simulink model "DACS"  (R2022b)
settings: Solver=VariableStepAuto  StartTime=0.0  StopTime=10  RelTol=1e-3
InitFcn:
  | DACSpara
values from neighbouring files (symbols this model uses):
  Amax = 362.97    [DACSpara.m]
  Dmax = 5415.1    [DACSpara.m]
  g = 9.52    [DACSpara.m]
  Ixx = M*(ly^2)/2    (= 0.2997)    [DACSpara.m]
  Iyy = M*(3*ly^2+4*lx^2)/12    (= 82.3052666667)    [DACSpara.m]
  Izz = M*(3*ly^2+4*lx^2)/12    (= 82.3052666667)    [DACSpara.m]
  Kd = 400    [Controlgain.m]    (also in DACSpara.m)
  Kp = 600    [Controlgain.m]    (also in DACSpara.m)
  Kp1 = 600    [Controlgain.m]    (also in DACSpara.m)
  Kp2 = 150    [Controlgain.m]    (also in DACSpara.m)
  lx = 1.825    [DACSpara.m]
  ly = 0.09    [DACSpara.m]
  M = 74    [DACSpara.m]
  N = 3    [Controlgain.m]    (also in DACSpara.m = 5)
  POSinit = [0; 0; 0]    [DACSpara.m]
  PQRinit = [0; 0; 0]    [DACSpara.m]
  Quatinit = Euler2Quat([phi;theta;psi].*d2r)    [DACSpara.m]
  Theading = Euler2Quat([0;-30;180].*d2r)    [DACSpara.m]
  TPosition = 20000*[Tpos(2);Tpos(3);-Tpos(4)]    [DACSpara.m]    (also in Targetpara.m = Tdist*[Tpos(2);Tpos(3);-Tpos(4)])
  Tspeed = 2500    [DACSpara.m]
  UVWinit = [1000; 0; 0]    [DACSpara.m]
libraries: matrix_library x2, dspmtrx3 x1, uavutilslib x1
settings Model: PacingRate=0.010000  Creator=tn  LastModifiedBy=tn
settings DataIOCC: ReturnWorkspaceOutputs=off

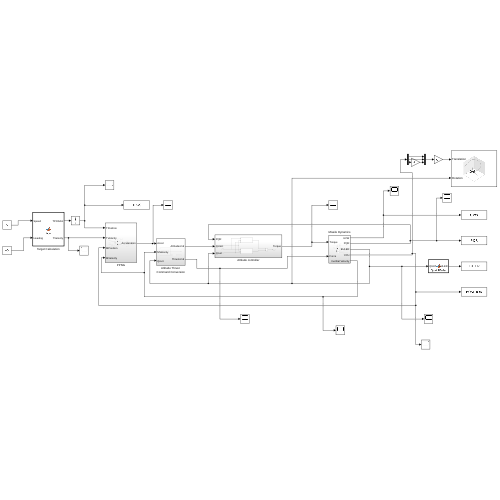
[thumbnail: Simulink's stored preview of the top-level diagram]
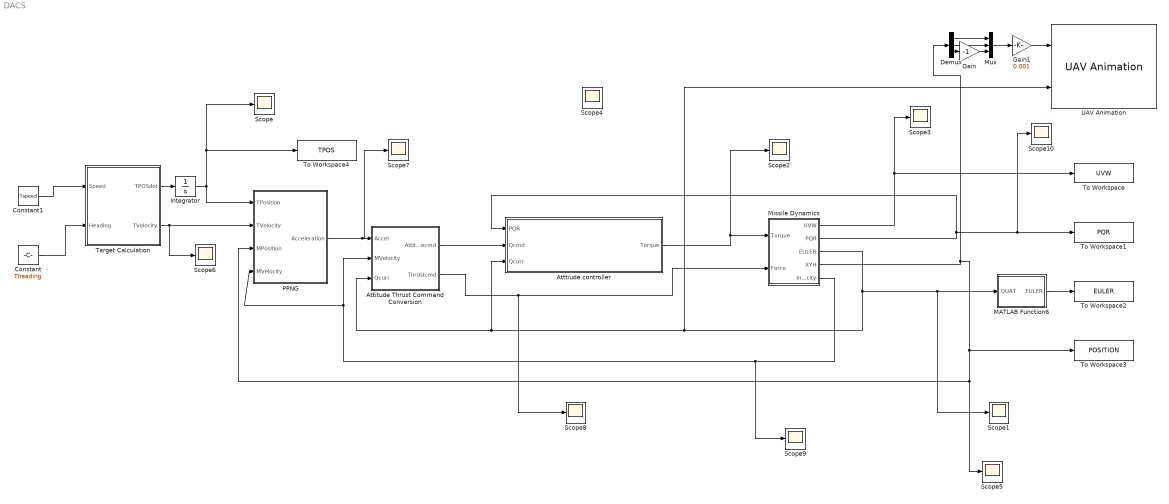
== system DACS ==
  Attitude Thrust Command Conversion : Subsystem
  Atttiude controller : Subsystem
  Constant : Constant  Value=Theading
  Constant1 : Constant  Value=Tspeed
  Demux : Demux  Outputs=3
  Gain : Gain  Gain=-1
  Gain1 : Gain  Gain=0.001
  Integrator : Integrator  InitialCondition=TPosition
  MATLAB Function6 : MATLAB Function  TreatAsAtomicUnit=on
  Missile Dynamics : Subsystem
  Mux : Mux  Inputs=3
  PPNG : Subsystem
  Scope{,1..10} (11 alike) : Scope
  Target Calculation : MATLAB Function  TreatAsAtomicUnit=on
  To Workspace : ToWorkspace  VariableName=UVW  SaveFormat=Timeseries  SampleTime=-1
  To Workspace1 : ToWorkspace  VariableName=PQR  SaveFormat=Timeseries  SampleTime=-1
  To Workspace2 : ToWorkspace  VariableName=EULER  SaveFormat=Timeseries  SampleTime=-1
  To Workspace3 : ToWorkspace  VariableName=POSITION  SaveFormat=Timeseries  SampleTime=-1
  To Workspace4 : ToWorkspace  VariableName=TPOS  SaveFormat=Timeseries  SampleTime=-1
  UAV Animation : uavutilslib/UAV Animation  UAVType=FixedWing  UAVSize=1  InertialZDirection=Down  SampleTime=-1
  wires:
  Missile Dynamics/1(UVW) -> To Workspace/1, Scope3/1
  Missile Dynamics/4(XYH) -> Demux/1, Scope5/1, PPNG/3(MPosition), To Workspace3/1
  Missile Dynamics/2(PQR) -> Atttiude controller/1(PQR), Scope10/1, To Workspace1/1
  Atttiude controller/1(Torque) -> Scope2/1, Missile Dynamics/1(Torque)
  Missile Dynamics/3(EULER) -> Atttiude controller/3(Qcurr), Attitude Thrust Command Conversion/3(Qcurr), UAV Animation/2, MATLAB Function6/1(QUAT), Scope1/1
  Missile Dynamics/5(Inerttial Velocity) -> Scope9/1, Attitude Thrust Command Conversion/2(MVelocity), PPNG/4(MVelocity)
  PPNG/1(Acceleration) -> Scope7/1, Attitude Thrust Command Conversion/1(Accel)
  Attitude Thrust Command Conversion/1(Attitudecmd) -> Atttiude controller/2(Qcmd)
  MATLAB Function6/1(EULER) -> To Workspace2/1
  Attitude Thrust Command Conversion/2(Thrustcmd) -> Scope8/1, Missile Dynamics/2(Force)
  Target Calculation/2(TVelocity) -> Scope6/1, PPNG/2(TVelocity)
  Integrator/1 -> Scope/1, To Workspace4/1, PPNG/1(TPosition)
  Constant1/1 -> Target Calculation/1(Speed)
  Constant/1 -> Target Calculation/2(Heading)
  Demux/1 -> Mux/1
  Demux/2 -> Mux/2
  Demux/3 -> Gain/1
  Gain/1 -> Mux/3
  Target Calculation/1(TPOSdot) -> Integrator/1
  Mux/1 -> Gain1/1
  Gain1/1 -> UAV Animation/1

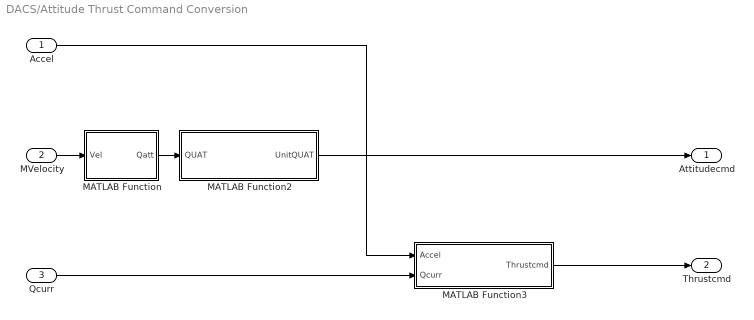
== system DACS/Attitude Thrust Command Conversion ==
  Accel : Inport
  MVelocity : Inport  Port=2
  Qcurr : Inport  Port=3
  MATLAB Function : MATLAB Function  TreatAsAtomicUnit=on
  MATLAB Function2 : MATLAB Function  TreatAsAtomicUnit=on
  MATLAB Function3 : MATLAB Function  TreatAsAtomicUnit=on
  Attitudecmd : Outport
  Thrustcmd : Outport  Port=2
  wires:
  MATLAB Function/1(Qatt) -> MATLAB Function2/1(QUAT)
  MVelocity/1 -> MATLAB Function/1(Vel)
  MATLAB Function2/1(UnitQUAT) -> Attitudecmd/1
  Qcurr/1 -> MATLAB Function3/2(Qcurr)
  Accel/1 -> MATLAB Function3/1(Accel)
  MATLAB Function3/1(Thrustcmd) -> Thrustcmd/1

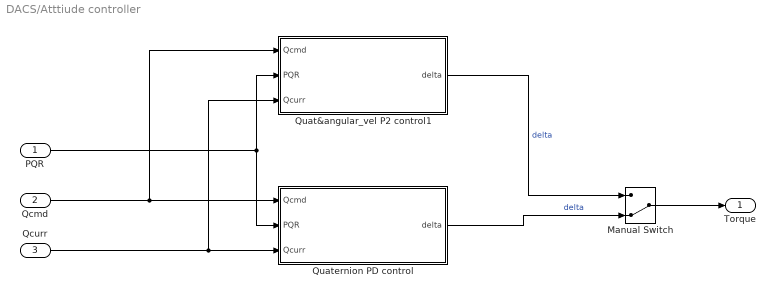
== system DACS/Atttiude controller ==
  PQR : Inport
  Qcmd : Inport  Port=2
  Qcurr : Inport  Port=3
  Manual Switch : ManualSwitch  CurrentSetting=0
  Quat&angular_vel P2 control1 : Subsystem
  Quaternion PD control : Subsystem
  Torque : Outport
  wires:
  Quaternion PD control/1(delta) -> Manual Switch/2  "delta"
  Quat&angular_vel P2 control1/1(delta) -> Manual Switch/1  "delta"
  Qcurr/1 -> Quaternion PD control/3(Qcurr), Quat&angular_vel P2 control1/3(Qcurr)
  Manual Switch/1 -> Torque/1
  Qcmd/1 -> Quaternion PD control/1(Qcmd), Quat&angular_vel P2 control1/1(Qcmd)
  PQR/1 -> Quat&angular_vel P2 control1/2(PQR), Quaternion PD control/2(PQR)

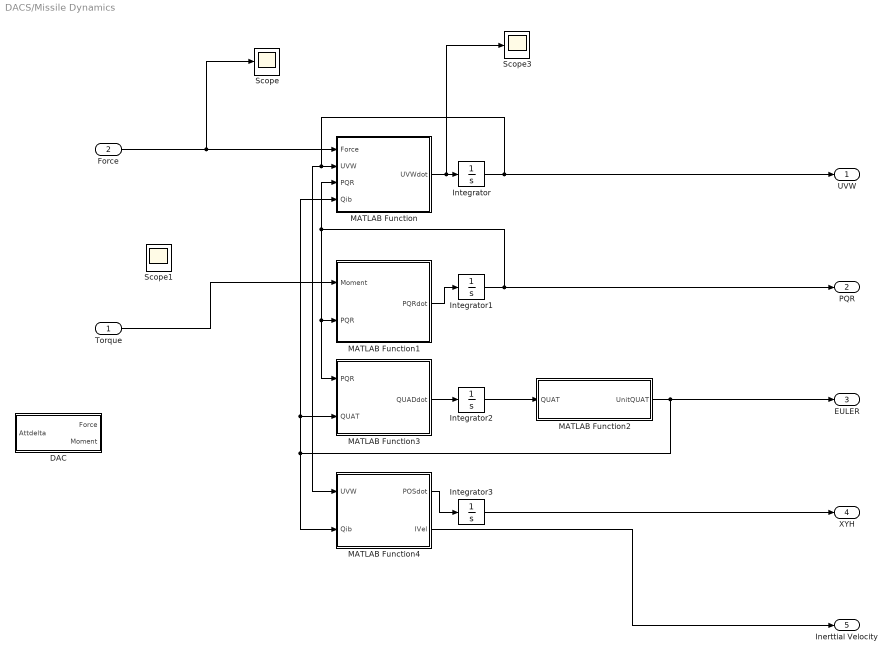
== system DACS/Missile Dynamics ==
  Torque : Inport
  Force : Inport  Port=2
  DAC : Subsystem
  Integrator : Integrator  InitialCondition=UVWinit
  Integrator1 : Integrator  InitialCondition=PQRinit
  Integrator2 : Integrator  InitialCondition=Quatinit
  Integrator3 : Integrator  InitialCondition=POSinit
  MATLAB Function : MATLAB Function  TreatAsAtomicUnit=on
  MATLAB Function1 : MATLAB Function  TreatAsAtomicUnit=on
  MATLAB Function2 : MATLAB Function  TreatAsAtomicUnit=on
  MATLAB Function3 : MATLAB Function  TreatAsAtomicUnit=on
  MATLAB Function4 : MATLAB Function  TreatAsAtomicUnit=on
  Scope : Scope
  Scope1 : Scope
  Scope3 : Scope
  UVW : Outport
  PQR : Outport  Port=2
  EULER : Outport  Port=3
  XYH : Outport  Port=4
  Inerttial Velocity : Outport  Port=5
  wires:
  MATLAB Function/1(UVWdot) -> Scope3/1, Integrator/1
  MATLAB Function1/1(PQRdot) -> Integrator1/1
  MATLAB Function3/1(QUADdot) -> Integrator2/1
  MATLAB Function4/1(POSdot) -> Integrator3/1
  Integrator/1 -> UVW/1, MATLAB Function4/1(UVW), MATLAB Function/2(UVW)
  Integrator1/1 -> PQR/1, MATLAB Function3/1(PQR), MATLAB Function1/2(PQR), MATLAB Function/3(PQR)
  Integrator2/1 -> MATLAB Function2/1(QUAT)
  MATLAB Function2/1(UnitQUAT) -> EULER/1, MATLAB Function4/2(Qib), MATLAB Function/4(Qib), MATLAB Function3/2(QUAT)
  Integrator3/1 -> XYH/1
  Torque/1 -> MATLAB Function1/1(Moment)
  Force/1 -> Scope/1, MATLAB Function/1(Force)
  MATLAB Function4/2(IVel) -> Inerttial Velocity/1

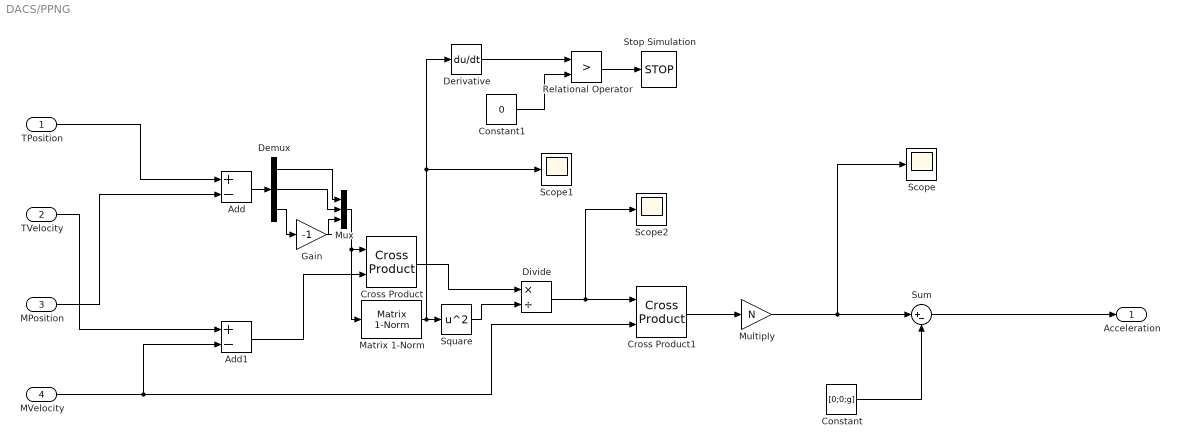
== system DACS/PPNG ==
  TPosition : Inport
  TVelocity : Inport  Port=2
  MPosition : Inport  Port=3
  MVelocity : Inport  Port=4
  Add : Sum  Inputs=+-
  Add1 : Sum  Inputs=+-
  Constant : Constant  Value=[0;0;g]
  Constant1 : Constant  Value=0
  Cross Product : matrix_library/Cross Product
  Cross Product1 : matrix_library/Cross Product
  Demux : Demux  Outputs=3
  Derivative : Derivative
  Divide : Product  Inputs=*/
  Gain : Gain  Gain=-1
  Matrix 1-Norm : dspmtrx3/Matrix  1-Norm  roundingMode=Floor  overflowMode=off  outputDataTypeStr=Inherit: Same as accumulator  outputMin=[]  outputMax=[]  outputLastDataTypeStr=Inherit: Same as accumulator
  Multiply : Gain  Gain=N
  Mux : Mux  Inputs=3
  Relational Operator : RelationalOperator  Operator=>  OutDataTypeStr=boolean  RndMeth=Simplest  InputSameDT=off
  Scope : Scope
  Scope1 : Scope
  Scope2 : Scope
  Square : Math  Operator=square
  Stop Simulation : Stop
  Sum : Sum  Inputs=|+-
  Acceleration : Outport
  wires:
  MPosition/1 -> Add/2
  TVelocity/1 -> Add1/1
  MVelocity/1 -> Cross Product1/2, Add1/2
  Add/1 -> Demux/1
  Add1/1 -> Cross Product/2
  Cross Product/1 -> Divide/1
  Divide/1 -> Scope2/1, Cross Product1/1
  Cross Product1/1 -> Multiply/1
  Multiply/1 -> Scope/1, Sum/1
  Constant/1 -> Sum/2
  Sum/1 -> Acceleration/1
  Square/1 -> Divide/2
  Matrix 1-Norm/1 -> Derivative/1, Scope1/1, Square/1
  Demux/3 -> Gain/1
  Constant1/1 -> Relational Operator/2
  TPosition/1 -> Add/1
  Demux/1 -> Mux/1
  Demux/2 -> Mux/2
  Gain/1 -> Mux/3
  Mux/1 -> Matrix 1-Norm/1, Cross Product/1
  Derivative/1 -> Relational Operator/1
  Relational Operator/1 -> Stop Simulation/1

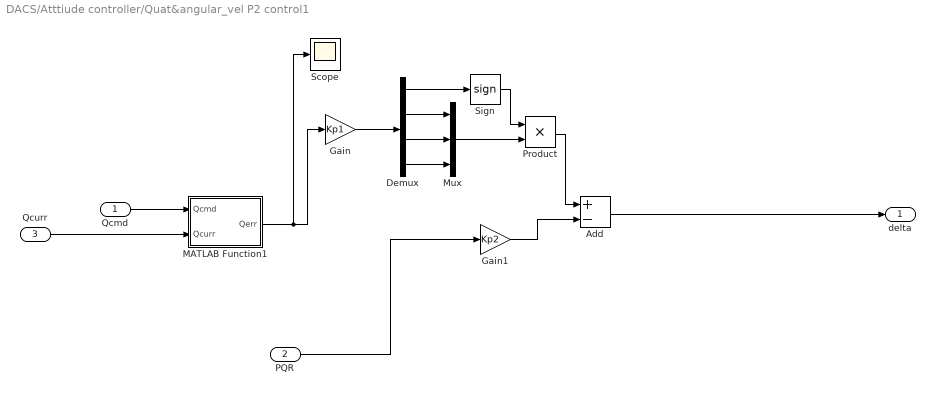
== system DACS/Atttiude controller/Quat&angular_vel P2 control1 ==
  Qcmd : Inport
  PQR : Inport  Port=2
  Qcurr : Inport  Port=3
  Add : Sum  Inputs=+-
  Demux : Demux
  Gain : Gain  Gain=Kp1
  Gain1 : Gain  Gain=Kp2
  MATLAB Function1 : MATLAB Function  TreatAsAtomicUnit=on
  Mux : Mux  Inputs=3
  Product : Product
  Scope : Scope
  Sign : Signum
  delta : Outport
  wires:
  Demux/3 -> Mux/2
  Demux/2 -> Mux/1
  MATLAB Function1/1(Qerr) -> Scope/1, Gain/1
  Gain1/1 -> Add/2
  PQR/1 -> Gain1/1
  Demux/4 -> Mux/3
  Qcurr/1 -> MATLAB Function1/2(Qcurr)
  Qcmd/1 -> MATLAB Function1/1(Qcmd)
  Gain/1 -> Demux/1
  Add/1 -> delta/1
  Demux/1 -> Sign/1
  Mux/1 -> Product/2
  Sign/1 -> Product/1
  Product/1 -> Add/1

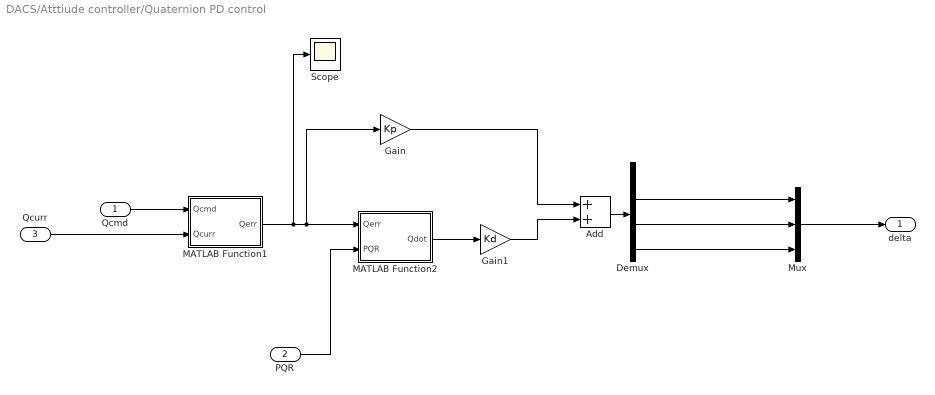
== system DACS/Atttiude controller/Quaternion PD control ==
  Qcmd : Inport
  PQR : Inport  Port=2
  Qcurr : Inport  Port=3
  Add : Sum
  Demux : Demux
  Gain : Gain  Gain=Kp
  Gain1 : Gain  Gain=Kd
  MATLAB Function1 : MATLAB Function  TreatAsAtomicUnit=on
  MATLAB Function2 : MATLAB Function  TreatAsAtomicUnit=on
  Mux : Mux  Inputs=3
  Scope : Scope
  delta : Outport
  wires:
  Demux/3 -> Mux/2
  PQR/1 -> MATLAB Function2/2(PQR)
  Demux/2 -> Mux/1
  Gain/1 -> Add/1
  MATLAB Function1/1(Qerr) -> Scope/1, Gain/1, MATLAB Function2/1(Qerr)
  Gain1/1 -> Add/2
  Add/1 -> Demux/1
  MATLAB Function2/1(Qdot) -> Gain1/1
  Demux/4 -> Mux/3
  Qcurr/1 -> MATLAB Function1/2(Qcurr)
  Qcmd/1 -> MATLAB Function1/1(Qcmd)
  Mux/1 -> delta/1

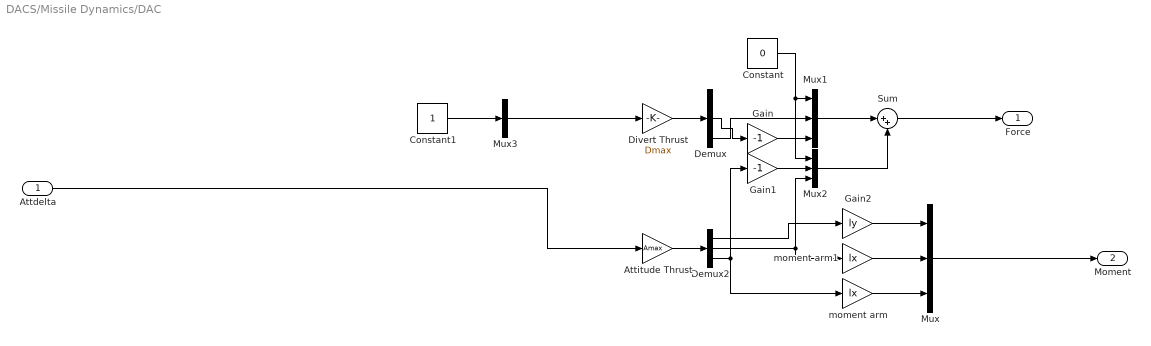
== system DACS/Missile Dynamics/DAC ==
  Attdelta : Inport
  Attitude Thrust : Gain  Gain=Amax
  Constant : Constant  Value=0
  Constant1 : Constant
  Demux : Demux  Outputs=3
  Demux2 : Demux  Outputs=3
  Divert Thrust : Gain  Gain=Dmax
  Gain : Gain  Gain=-1
  Gain1 : Gain  Gain=-1
  Gain2 : Gain  Gain=ly
  Mux{,1..3} (4 alike) : Mux  Inputs=3
  Sum : Sum  Inputs=|++
  moment arm : Gain  Gain=lx
  moment arm1 : Gain  Gain=lx
  Force : Outport
  Moment : Outport  Port=2
  wires:
  Attitude Thrust/1 -> Demux2/1
  Sum/1 -> Force/1
  Mux1/1 -> Sum/1
  Demux2/1 -> Gain2/1
  Gain/1 -> Mux1/3
  Demux2/3 -> moment arm/1, Gain1/1
  Gain1/1 -> Mux2/2
  Demux2/2 -> moment arm1/1, Mux2/3
  Mux2/1 -> Sum/2
  Mux/1 -> Moment/1
  Constant/1 -> Mux1/1, Mux2/1
  Divert Thrust/1 -> Demux/1
  Demux/3 -> Mux1/2
  Demux/2 -> Gain/1
  Gain2/1 -> Mux/1
  moment arm1/1 -> Mux/2
  moment arm/1 -> Mux/3
  Attdelta/1 -> Attitude Thrust/1
  Constant1/1 -> Mux3/2
  Mux3/1 -> Divert Thrust/1

== matlab function DACS/Attitude Thrust Command Conversion/MATLAB Function ==
  data: Vel input; Qatt output
function Qatt = fcn(Vel)

if (nnz(Vel./norm(Vel) == -[1;0;0]) == 3)
    Qatt = [0;0;1;0];
    return
end

temp = cross([1;0;0],Vel);
q0 = norm(Vel)+dot(Vel,[1;0;0]);

Qatt = [q0;temp(1);temp(2);temp(3)];
end

== matlab function DACS/Attitude Thrust Command Conversion/MATLAB Function3 ==
  data: Accel input; Thrustcmd output; Qcurr input; Dmax parameter; M parameter
function Thrustcmd   = Projection(Accel, Qcurr, Dmax,M)

temp = Quatmul(Quatmul(Quatinv(Qcurr),Accel),Qcurr);
Thrustcmd = M.*[0;temp(3);temp(4)];
if (norm(Thrustcmd) > Dmax)
    Thrustcmd = Dmax*Thrustcmd./norm(Thrustcmd);
end

== matlab function DACS/Attitude Thrust Command Conversion/MATLAB Function2 ==
  data: QUAT input; UnitQUAT output
function UnitQUAT = NormalizeQuat(QUAT)

q0 = QUAT(1);
q1 = QUAT(2);
q2 = QUAT(3);
q3 = QUAT(4);

Qabs = sqrt(q0^2+q1^2+q2^2+q3^2);

q0 = q0/Qabs;
q1 = q1/Qabs;
q2 = q2/Qabs;
q3 = q3/Qabs;

UnitQUAT = [q0;q1;q2;q3];
end

== matlab function DACS/Missile Dynamics/MATLAB Function1 ==
  data: Moment input; PQRdot output; PQR input; Ixx parameter; Iyy parameter; Izz parameter
function PQRdot = PQR_dot(Moment, PQR, Ixx, Iyy, Izz)

p = PQR(1);
q = PQR(2);
r = PQR(3);

% L=0, So p_dot is zero, p is constant value
L = Moment(1);
M = Moment(2);
N = Moment(3);

p_dot = L/Ixx - (Izz-Iyy)*q*r/Ixx;
q_dot = M/Iyy - (Ixx-Izz)*p*r/Iyy;
r_dot = N/Izz - (Iyy-Ixx)*p*q/Izz;

PQRdot = [p_dot;q_dot;r_dot];

== matlab function DACS/Missile Dynamics/MATLAB Function ==
  data: Force input; UVWdot output; UVW input; PQR input; Qib input; M parameter
function UVWdot= UVW_dot(Force,UVW,PQR,Qib,M)

g=9.52;   % gravity @ 100km height [m/s^2]

fx = Force(1);
fy = Force(2);
fz = Force(3);

u = UVW(1);
v = UVW(2);
w = UVW(3);

p = PQR(1);
q = PQR(2);
r = PQR(3);

%gb = Cib'*[0; 0; g];
gcal = Quatmul(Quatmul(Quatinv(Qib),[0;0;g]), Qib);
gb = [gcal(2);gcal(3);gcal(4)];

u_dot = v*r - w*q + fx/M + gb(1);
v_dot = -u*r + w*p + fy/M + gb(2);
w_dot = u*q - v*p + fz/M + gb(3);

UVWdot =[u_dot; v_dot; w_dot];

== matlab function DACS/Missile Dynamics/MATLAB Function3 ==
  data: PQR input; QUAT input; QUADdot output
function QUADdot = QUAT_dot(PQR,QUAT)

q0 = QUAT(1);
q1 = QUAT(2);
q2 = QUAT(3);
q3 = QUAT(4);

p = PQR(1);
q = PQR(2);
r = PQR(3);
    
q0_dot = -1/2*(q1*p +q2*q + q3*r);
q1_dot = 1/2*(q0*p +q2*r - q3*q);
q2_dot = 1/2*(q0*q +q3*p - q1*r);
q3_dot = 1/2*(q0*r +q1*q - q2*p);

QUADdot =[q0_dot; q1_dot; q2_dot; q3_dot];

== matlab function DACS/Missile Dynamics/MATLAB Function4 ==
  data: POSdot output; IVel output; UVW input; Qib input
function [POSdot, IVel] = POS_dot(UVW,Qib)

u = UVW(1);
v = UVW(2);
w = UVW(3);

POSdotcal = Quatmul(Quatmul(Qib,[u; v; w]), Quatinv(Qib));
IVel = [POSdotcal(2);POSdotcal(3);POSdotcal(4)];
POSdot = [1 0 0;0 1 0;0 0 -1]*IVel; % pos=[x,y,h]'

== matlab function DACS/Missile Dynamics/MATLAB Function2 ==
  data: QUAT input; UnitQUAT output
function UnitQUAT = NormalizeQuat(QUAT)

q0 = QUAT(1);
q1 = QUAT(2);
q2 = QUAT(3);
q3 = QUAT(4);

Qabs = sqrt(q0^2+q1^2+q2^2+q3^2);

q0 = q0/Qabs;
q1 = q1/Qabs;
q2 = q2/Qabs;
q3 = q3/Qabs;

UnitQUAT = [q0;q1;q2;q3];
end

== matlab function DACS/Atttiude controller/Quat&angular_vel P2 control1/MATLAB Function1 ==
  data: Qcmd input; Qerr output; Qcurr input
function Qerr = ErrorQ(Qcmd, Qcurr)

qx = Quatinv(Qcurr);

Qerr = Quatmul(qx, Qcmd);
end

== matlab function DACS/MATLAB Function6 ==
  data: QUAT input; EULER output
function EULER = Quat2Euler(QUAT)

q0 = QUAT(1);
q1 = QUAT(2);
q2 = QUAT(3);
q3 = QUAT(4);

phi = atan2(2*(q0*q1+q2*q3), (q0^2+q3^2-q1^2-q2^2));
theta = asin(2*(q0*q2-q1*q3));
psi = atan2(2*(q1*q2+q0*q3), (q0^2+q1^2-q2^2-q3^2));

EULER = [phi; theta; psi];

== matlab function DACS/Target Calculation ==
  data: TPOSdot output; Speed input; Heading input; TVelocity output
function [TPOSdot, TVelocity]  = fcn(Speed, Heading)

temp = Quatmul(Quatmul(Heading,[Speed;0;0]),Quatinv(Heading));
TVelocity = [temp(2);temp(3);temp(4)];
TPOSdot = [1 0 0;0 1 0;0 0 -1] * TVelocity; % [X;Y;H]
end

== matlab function DACS/Atttiude controller/Quaternion PD control/MATLAB Function1 ==
  data: Qcmd input; Qerr output; Qcurr input
function Qerr = ErrorQ(Qcmd, Qcurr)

qx = Quatinv(Qcurr);

Qerr = Quatmul(qx, Qcmd);
end

== matlab function DACS/Atttiude controller/Quaternion PD control/MATLAB Function2 ==
  data: Qerr input; Qdot output; PQR input
function Qdot = DeriveQ(Qerr, PQR)

q0 = Qerr(1);
q1 = Qerr(2);
q2 = Qerr(3);
q3 = Qerr(4);

p = PQR(1);
q = PQR(2);
r = PQR(3);

%qx = [q0 -q1 -q2 -q3; q1 q0 -q3 q2; q2 q3 q0 -q1; q3 -q2 q1 q0];
PQRquat = [0;p;q;r];

Qdot = -1/2.*Quatmul(PQRquat,Qerr);
end
